simulink model "three_phase_csi_wihtout_pwm_technique"  (R2014a)
settings: Solver=ode45  StartTime=0.0  StopTime=1  RelTol=1e-3
libraries: powerlib x13, powerlib_meascontrol x2
settings Model: Creator=singa  LastModifiedBy=singa

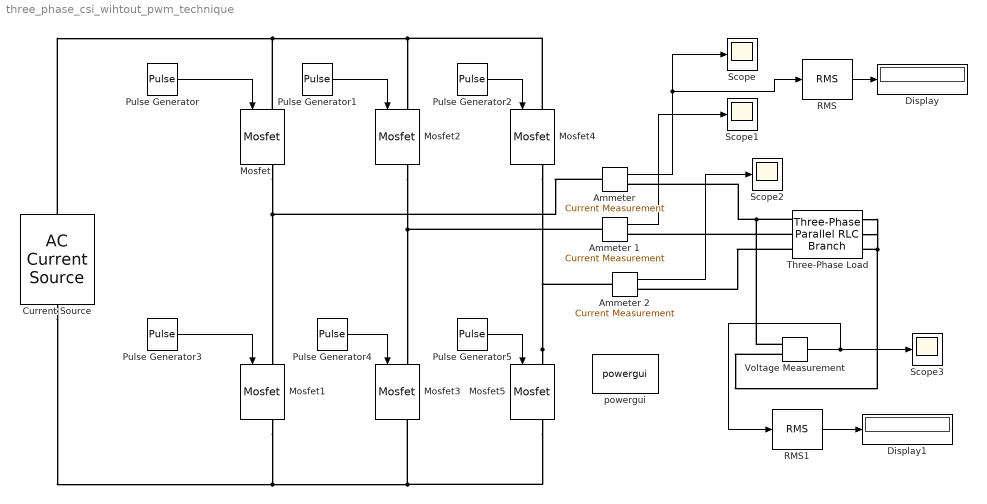
== system three_phase_csi_wihtout_pwm_technique ==
  Ammeter : powerlib/Measurements/Current Measurement  PhasorSimulation=off  OutputType=Complex  PSBequivalent=0
  Ammeter 1 : powerlib/Measurements/Current Measurement  PhasorSimulation=off  OutputType=Complex  PSBequivalent=0
  Ammeter 2 : powerlib/Measurements/Current Measurement  PhasorSimulation=off  OutputType=Complex  PSBequivalent=0
  Current Source : powerlib/Electrical Sources/AC Current Source  Amplitude=200  Phase=90  Frequency=0  SampleTime=0  Measurements=None
  Display : Display
  Display1 : Display
  Mosfet{,1..5} (6 alike) : powerlib/Power Electronics/Mosfet  Ron=0.1  Lon=0  Rd=0.01  Vfd=0  IC=0  Rs=1e5  Cs=inf  Measurements=on
  Pulse Generator : DiscretePulseGenerator  PulseType=Time based  Period=0.02  PulseWidth=50
  Pulse Generator1 : DiscretePulseGenerator  PulseType=Time based  Period=0.02  PulseWidth=50  PhaseDelay=0.02/3
  Pulse Generator2 : DiscretePulseGenerator  PulseType=Time based  Period=0.02  PulseWidth=50  PhaseDelay=0.04/3
  Pulse Generator3 : DiscretePulseGenerator  PulseType=Time based  Period=0.02  PulseWidth=50  PhaseDelay=0.01
  Pulse Generator4 : DiscretePulseGenerator  PulseType=Time based  Period=0.02  PulseWidth=50  PhaseDelay=0.01+0.02/3
  Pulse Generator5 : DiscretePulseGenerator  PulseType=Time based  Period=0.02  PulseWidth=50  PhaseDelay=0.01+0.04/3
  RMS : powerlib_meascontrol/Measurements/RMS  TrueRMS=on  Freq=50  RMSInit=120  Ts=0
  RMS1 : powerlib_meascontrol/Measurements/RMS  TrueRMS=on  Freq=50  RMSInit=120  Ts=0
  Scope{,1..3} (4 alike) : Scope
      Scope settings: YMin=-8  YMax=8  SampleInput=on  SampleTime=1e-6
      Scope1 settings: YMin=-8  YMax=8  SampleInput=on  SampleTime=1e-6
      Scope2 settings: YMin=-8  YMax=8  SaveName=ScopeData2  SampleInput=on  SampleTime=1e-6
      Scope3 settings: YMin=-8  YMax=8  SaveName=ScopeData3  SampleInput=on  SampleTime=1e-6
  Three-Phase Load : powerlib/Elements/Three-Phase Parallel RLC Branch  LConnTagsString=A|B|C  RConnTagsString=A|B|C  BranchType=RC  Resistance=1  Inductance=1e-3  Capacitance=0.1  Measurements=None
  Voltage Measurement : powerlib/Measurements/Voltage Measurement  PhasorSimulation=off  OutputType=Complex  PSBequivalent=0
  powergui : powerlib/powergui  Priority=1  SimulationMode=Continuous  SolverType=Tustin  SampleTime=50e-6  frequency=60  SPID=off  DisableSnubberDevices=off  DisableRonSwitches=off  DisableVfSwitches=off  SwTol=0  Interpol=off  DisplayEquations=off  Ts=0  methode=off  frequencyindice=0  Pbase=100e6  ErrMax=1e-4  Iterations=50  UnitsV=kV  UnitsW=MW  FunctionMessages=off  echomessages=off  HookPort=off  EnableUseOfTLC=off  x0status=blocks  RestoreLinks=warning  ResistiveCurrentMeasurement=off  Frange=[0:2:500]  Ylog=off  Xlog=on  ShowGrid=off  save=off  variable=ZData  structure=ScopeData3  ZoomFFT=off  StartTime=0.8  cycles=2  DisplayStyle=4  fundamental=50  FreqAxis=on  MaxFrequency=2500  frequencyindicesteady=1  RmsSteady=1  display=off
  wires:
  Ammeter/1 -> Scope/1, RMS/1
  Ammeter 1/1 -> Scope1/1
  Ammeter 2/1 -> Scope2/1
  Pulse Generator/1 -> Mosfet/1
  Pulse Generator1/1 -> Mosfet2/1
  Pulse Generator2/1 -> Mosfet4/1
  Pulse Generator3/1 -> Mosfet1/1
  Pulse Generator4/1 -> Mosfet3/1
  Pulse Generator5/1 -> Mosfet5/1
  Voltage Measurement/1 -> RMS1/1, Scope3/1
  RMS/1 -> Display/1
  RMS1/1 -> Display1/1
  connections:
  Ammeter/LConn1 -- Mosfet/RConn1 -- Mosfet1/LConn1
  Ammeter 1/LConn1 -- Mosfet2/RConn1 -- Mosfet3/LConn1
  Mosfet5/LConn1 -- Mosfet4/RConn1 -- Ammeter 2/LConn1
  Current Source/RConn1 -- Mosfet/LConn1 -- Mosfet4/LConn1 -- Mosfet2/LConn1
  Current Source/LConn1 -- Mosfet1/RConn1 -- Mosfet5/RConn1 -- Mosfet3/RConn1
  Three-Phase Load/RConn1 -- Three-Phase Load/RConn2 -- Voltage Measurement/LConn2 -- Three-Phase Load/RConn3
  Three-Phase Load/LConn3 -- Ammeter 2/RConn1
  Three-Phase Load/LConn2 -- Ammeter 1/RConn1
  Three-Phase Load/LConn1 -- Voltage Measurement/LConn1 -- Ammeter/RConn1
